simulink model "Nanogrid"  (R2026a)
settings: Solver=VariableStepAuto  StopTime=3
PreLoadFcn:
  | NanogridParam
undefined symbols (not defined in the file): baseLoad, bessSystem, bessVoltage, DiscIntNeverNeededParam, ee_sli_rtmsupport, gcbh, gflInverter, gfmInverter, nanoLoad, PV, PVInverter, ref, solar, solarInsolationChange, Ts
libraries: nesl_utility x51, eeGeneralControl x38, ee_lib x33, fl_lib x24, simulink x20, eeTransforms x13, slpidlib x8, nesl_utility_internal x4, sl_signal_attributes x4, sl_discontinuities x4, eeSinusoidalMeasurementV2 x3, batteryecm_lib x2
(part 1 of 6)
settings Model: Creator=claude-test  LastModifiedBy=claude-test

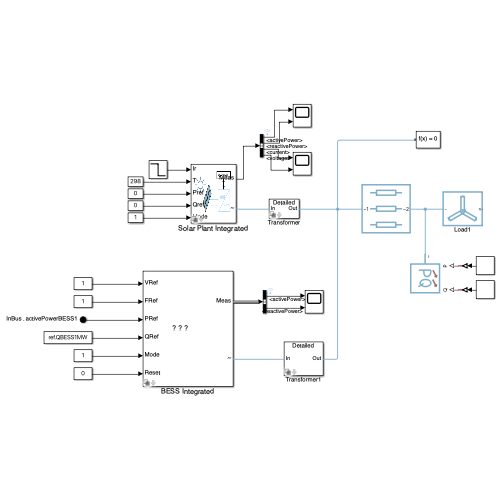
[thumbnail: Simulink's stored preview of the top-level diagram]
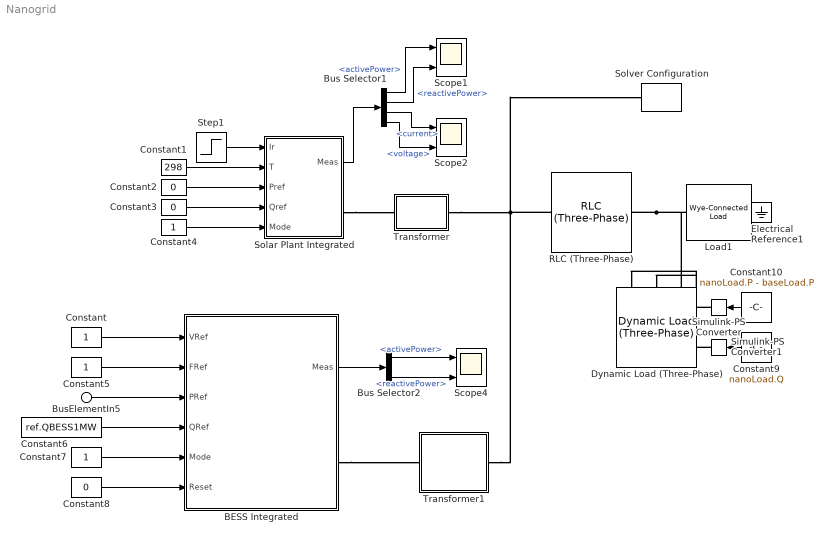
== system Nanogrid ==
  BusElementIn5 : Inport  PortName=InBus  Element=activePowerBESS1
  BESS Integrated : Subsystem  Variant=on  VariantControlMode=label  LabelModeActiveChoice=Detailed  mask(Battery Energy Storage System (BESS)){fidelity=Detailed, bessController=Grid Forming, plantRating=bessSystem.plantRating, Vac=bessSystem.Vac, frequency=bessSystem.frequency, iMaxPU=bessSystem.iMaxPU, efficiency=bessSystem.converterEfficiency, baseVoltageDC=bessSystem.Vdc, filterInductance=bessSystem.filterInductance, filterResistance=bessSystem.filterResistance, maxSOC=bessSystem.maxSOC, minSOC=bessSystem.minSOC, converterFidelity=Average, fSw=bessSystem.switchingFrequency, activeDroop=bessSystem.activeDroop, reactiveDroop=bessSystem.reactiveDroop, maxSOCGFM=0.95, minSOCGFM=0.1, initialSOC=bessSystem.initialSOC, capacityType=Infinite, capacity=1000}
      mask prompts: fidelity "Modeling Option"; bessController "Operating Mode"; plantRating "BESS Rating (kW)"; Vac "Rated AC side voltage (phase-phase RMS) (V)"; frequency "Rated electrical frequency at AC side (Hz)"; iMaxPU "Maximum converter current (pu)"; efficiency "Converter Efficiency (%)"; baseVoltageDC "Voltage on DC side (V)"; filterInductance "Filter inductance (H)"; filterResistance "Filter series resistance (Ohm)"; maxSOC "Maximum  operating SOC"; minSOC "Minimum  operating SOC"; converterFidelity "Converter Fidelity"; fSw "Switching Frequency (kHz)"; activeDroop "Active droop"; reactiveDroop "Reactive droop"; maxSOCGFM "Maximum  operating SOC"; minSOCGFM "Minimum  operating SOC"; initialSOC "Initial SOC"; capacityType "Battery charge capacity"; capacity "Battery capacity (Ah)"
      mask help:
      | This block represents a flexible BESS that can be configured for different operational modes and modeling fidelities. It supports Grid-Following (GFL) and Grid-Forming (GFM) control strategies, along with two fidelity levels:
      |
      | Detailed – captures dynamic control loops and converter behavior for accurate transient analysis.
      | Simplified – optimized for faster simulations while preserving essential system characteristics.
      settings: CopyFcn=set_param(gcbh,'LinkStatus','none');
      mask Help: web('BESS.html')
      mask TypeOptions fidelity: Detailed | Simplified
      mask Callback fidelity:
      | component.mask.fidelitySelection;
      |     fidelity = get_param(gcb,'fidelity');
      |     mode = get_param(gcb,'bessController');
      |     maskObj = Simulink.Mask.get(gcb);
      |     allNames = {maskObj.Parameters.Name};
      |     effIdx = find(strcmp(allNames, 'efficiency'));
      |     tabGFL = maskObj.getDialogControl('cellSimplified');
      |     tabGFM = maskObj.getDialogControl('cellSimplifiedGFM');
      |     if strcmp(fidelity,'Simplified')
      |         maskObj.Parameters(effIdx).Visible = 'on';
      |         if strcmp(mode,'Grid Following')
      |             tabGFL.Visible = 'on';
      |             tabGFM.Visible = 'off';
      |         else
      |             tabGFL.Visible = 'off';
      |             tabGFM.Visible = 'on';
      |         end
      |     else
      |         maskObj.Parameters(effIdx).Visible = 'off';
      |         tabGFL.Visible = 'off';
      |         tabGFM.Visible = 'off';
      |     end
      mask TypeOptions bessController: Grid Following | Grid Forming
      mask Callback bessController:
      | fidelity = get_param(gcb,'fidelity');
      | mode = get_param(gcb,'bessController');
      | if strcmp(fidelity,'Detailed')
      |     component.mask.setBESSController;
      | else
      |     blockPath = [gcb,'/','Simplified'];
      |     component.mask.setBESSController(blockPath);
      | end
      | maskObj = Simulink.Mask.get(gcb);
      | tabGFL = maskObj.getDialogControl('cellSimplified');
      | tabGFM = maskObj.getDialogControl('cellSimplifiedGFM');
      | if strcmp(fidelity,'Simplified')
      |     if strcmp(mode,'Grid Following')
      |         tabGFL.Visible = 'on';
      |         tabGFM.Visible = 'off';
      |     else
      |         tabGFL.Visible = 'off';
      |         tabGFM.Visible = 'on';
      |     end
      | else
      |     tabGFL.Visible = 'off';
      |     tabGFM.Visible = 'off';
      | end
      mask TypeOptions converterFidelity: Detailed/BESS Plant/converterFidelity
      mask Callback converterFidelity:
      | blockPath = [gcb,'/','Detailed','/','BESS Plant','/','Converter'];
      | component.mask.converterFidelity(blockPath);
      mask TypeOptions fSw: Detailed/PV Plant & Controller/PV Plant/fSw
      mask TypeOptions initialSOC: Simplified/Grid Forming/initialSOC
      mask TypeOptions capacityType: Simplified/Grid Forming/capacityType
      mask Callback capacityType: component.mask.configureBatteryCapacity;
      mask TypeOptions capacity: Simplified/Grid Forming/capacity
      mask DialogControl generalDetailed Prompt: General
      mask DialogControl cellDetailed Prompt: Battery
      mask DialogControl configureBattery Prompt: Edit battery parameters
      mask DialogControl configureBattery Callback:
      | blockPath = [gcb,'/','Detailed','/','BESS Plant','/','Battery'] ;
      |     component.mask.openBlock(blockPath);
      mask DialogControl controllerDetailed Prompt: BESS Controller
      mask DialogControl configureBESSController Prompt: Edit BESS Controller
      mask DialogControl configureBESSController Callback:
      | controllerType = get_param(gcb,'bessController');
      |     blockPath = [gcb,'/','Detailed','/','BESS Controller','/',controllerType];
      |     component.mask.openBlock(blockPath);
      mask DialogControl cellSimplified Prompt: Battery
      mask DialogControl configureBatterySimplified Prompt: Edit battery parameters
      mask DialogControl configureBatterySimplified Callback:
      | mode = get_param(gcb,'bessController');
      |     blockPath = [gcb,'/','Simplified','/',mode,'/','Battery'] ;
      |     if strcmp(mode,'Grid Following')
      |         component.mask.openBlock(blockPath);
      |     end
      mask DialogControl converter Prompt: Converter
      mask DialogControl editConverter Prompt: Edit converter parameters
      mask DialogControl editConverter Callback:
      | converterFidelity = get_param(gcb,'converterFidelity');
      | blockPath = [gcb,'/','Detailed','/','BESS Plant','/','Converter','/',converterFidelity,'/','Converter'];
      | component.mask.openBlock(blockPath);
      mask DialogControl cellSimplifiedGFM Prompt: Battery
      mask Display: image('battery_detailed.png');
  Bus Selector1 : BusSelector  OutputSignals=activePower,reactivePower,current,voltage
  Bus Selector2 : BusSelector  OutputSignals=activePower,reactivePower
  Constant{,4..5,7} (4 alike) : Constant
  Constant1 : Constant  Value=298
  Constant10 : Constant  Value=nanoLoad.P - baseLoad.P
  Constant2 : Constant  Value=0
  Constant3 : Constant  Value=0
  Constant6 : Constant  Value=ref.QBESS1MW
  Constant8 : Constant  Value=0
  Constant9 : Constant  Value=nanoLoad.Q
  Dynamic Load (Three-Phase) : ee_lib/Passive/Dynamic Load (Three-Phase)  port_option=ee.enum.threePhasePort.composite  FRated=systemFrequency Hz  Vline_rms_min=7700 V  tau=0.0167 s  Vline_rms_ini=11000 V  Vang_ini=0 deg  gmin=0 S
  Electrical Reference1 : fl_lib/Electrical/Electrical Elements/Electrical Reference
  Load1 : ee_lib/Passive/RLC Assemblies/Wye-Connected Load  port_option=ee.enum.threePhasePort.composite  parameterization=ee.enum.rlc.parameterization.ratedpower  component_structure=ee.enum.rlc.structure.R  component_structure_PQ=ee.enum.rlc.structure.R  R=1 Ohm  L=1e-3 H  C=1e-6 F  VRated=busVoltage V  FRated=systemFrequency Hz  P=baseLoad.P W  Qpos=0 A*V  Qneg=-1e2 A*V  R_parasitic=1e-6 Ohm  G_parasitic=1e-6 1/Ohm  R_parasitic_PQ=1e-6 Ohm  G_parasitic_PQ=1e-6 1/Ohm  Vmag0=busVoltage V  Vang0=0 deg  Freq0=systemFrequency Hz  IL_specify=off  IL_priority=High  IL=[0, 0, 0] A  IL_nominal_specify=off  IL_nominal_value=1  IL_nominal_unit=A  VC_specify=off  VC_priority=High  VC=[0, 0, 0] V  VC_nominal_specify=off  VC_nominal_value=1  VC_nominal_unit=V
  RLC (Three-Phase) : ee_lib/Passive/RLC Assemblies/RLC (Three-Phase)  port_option=ee.enum.threePhasePort.composite  component_structure=ee.enum.rlc.structure.SeriesRL  R=1 Ohm  L=1e-03 H  C=1e-6 F  R_parasitic=0 Ohm  G_parasitic=0 1/Ohm  IL_specify=off  IL_priority=High  IL=[0, 0, 0] A  IL_nominal_specify=off  IL_nominal_value=1  IL_nominal_unit=A  VC_specify=off  VC_priority=High  VC=[0, 0, 0] V  VC_nominal_specify=off  VC_nominal_value=1  VC_nominal_unit=V
  Scope1 : Scope  NumInputPorts=2
      settings: ActiveDisplayYMinimum=-0.88286408189414312  ActiveDisplayYMaximum=1.6939099105793236  DataLoggingVariableName=ScopeData17
  Scope2 : Scope  NumInputPorts=2
      settings: ActiveDisplayYMinimum=-0.88286408189414312  ActiveDisplayYMaximum=1.6939099105793236  DataLoggingVariableName=ScopeData18
  Scope4 : Scope  NumInputPorts=2
      settings: ActiveDisplayYMinimum=-0.88286408189414312  ActiveDisplayYMaximum=1.6939099105793236  DataLoggingVariableName=ScopeData55
  Simulink-PS Converter : nesl_utility/Simulink-PS Converter  PhysicalDomain=network_engine_domain  SubClassName=ps_input  LeftPortType=input  RightPortType=output  PseudoPeriodic=off  Frequencies=[]  NoiseDistribution=none  NoiseParameters=[]  Unit=1  AffineConversion=off  FilteringAndDerivatives=provide  SimscapeFilterOrder=1  InputFilterTimeConstant=0.001  UdotUserProvided=0
  Simulink-PS Converter1 : nesl_utility/Simulink-PS Converter  PhysicalDomain=network_engine_domain  SubClassName=ps_input  LeftPortType=input  RightPortType=output  PseudoPeriodic=off  Frequencies=[]  NoiseDistribution=none  NoiseParameters=[]  Unit=1  AffineConversion=off  FilteringAndDerivatives=provide  SimscapeFilterOrder=1  InputFilterTimeConstant=0.001  UdotUserProvided=0
  Solar Plant Integrated : Subsystem  Variant=on  VariantControlMode=label  LabelModeActiveChoice=Detailed  mask(Solar){fidelity=Detailed, plantRating=PV.plantRating, Vac=PV.Vac, frequency=PV.frequency, iMaxPU=PVInverter.iMaxPU, efficiency=PV.converterEfficiency, baseVoltageDC=PV.baseVoltageDC, nParallel=PV.nParallel, nSeries=30, capacitance=PVInverter.capacitance, filterInductance=PVInverter.filterInductance, filterResistance=PVInverter.filterResistance, panelType=Poly-crystalline, panelRating=PV.panelRating, Isc=PV.Isc, Voc=PV.Voc, irradianceSTC=PV.irradianceSTC, temperatureSTC=PV.temperatureSTC, alpha=PV.alpha, beta=PV.beta, mode=Maximum power point tracking, converterFidelity=Average, fSw=PV.switchingFrequency}
      mask prompts: fidelity "Modeling Option"; plantRating "Solar Plant Rating (kW)"; Vac "Rated AC side voltage (phase-phase RMS) (V)"; frequency "Rated electrical frequency at AC side (Hz)"; iMaxPU "Maximum converter current (pu)"; efficiency "Converter Efficiency (%)"; baseVoltageDC "Voltage on DC side (V)"; nParallel "Number of panels in parallel"; nSeries "Number of panels in series"; capacitance "DC bus capacitance (F)"; filterInductance "Filter inductance (H)"; filterResistance "Filter series resistance (Ohm)"; panelType "Panel Type"; panelRating "Panel Rating (W)"; Isc "Short-circuit current (A)"; Voc "Open-circuit voltage (V)"; irradianceSTC "Irradiance at STC (W/m² )"; temperatureSTC "Temperature at STC (°K)"; alpha "Temperature co-efficient for current (A/°K)"; beta "Temperature co-efficient for voltage (V/°K)"; mode "Operating Mode"; converterFidelity "Converter Fidelity"; fSw "Switching Frequency (kHz)"
      mask help: This block models a Solar PV plant. The detailed variant models MPPT, voltage and current controllers. The simplified variant is based on Anderson's translational equations. Select simplified mode for faster simulation using fixed efficiency and rated power.
      settings: CopyFcn=set_param(gcbh,'LinkStatus','none');
      mask Help: web('SolarPlant.html')
      mask TypeOptions fidelity: Detailed | Simplified
      mask Callback fidelity: component.mask.fidelitySelection;
      mask TypeOptions nParallel: Detailed/PV Plant & Controller/PV Plant/nParallel
      mask TypeOptions nSeries: Detailed/PV Plant & Controller/PV Plant/nSeries
      mask TypeOptions panelType: Poly-crystalline | Mono-crystalline | Cadmium-Telluride | Others
      mask Callback panelType: component.mask.selectSolarPanelType;
      mask TypeOptions mode: Maximum power point tracking | Power reference
      mask Callback mode:
      | % choice = get_param(gcb,'mode');
      | % blockPath = [gcb,'/','Solar','/','Simplified','/','Solar_Plant'];
      | % blockHandle = get_param(blockPath, 'Handle');
      | % if strcmp(choice,'Maximum power point tracking')
      | %     set_param(blockPath,'modelling_option','ModellingOption.maximumPower');
      | % else
      | %     set_param(blockPath,'modelling_option','ModellingOption.powerReference');
      | % end
      mask TypeOptions converterFidelity: Detailed/PV Plant & Controller/PV Plant/converterFidelity
      mask Callback converterFidelity: component.mask.setSwitchingFrequency;
      mask TypeOptions fSw: Detailed/PV Plant & Controller/PV Plant/fSw
      mask DialogControl generalDetailed Prompt: General
      mask DialogControl cellDetailed Prompt: Solar Cell
      mask DialogControl partsCatalog Prompt: Click to choose from parts catalog
      mask DialogControl partsCatalog Callback: component.mask.openParamManager;
      mask DialogControl panelCalculation Prompt: Calculate number of panels
      mask DialogControl panelCalculation Callback: component.mask.setPanelNumber;
      mask DialogControl configureSolarCell Prompt: Edit Solar Cell Parameters
      mask DialogControl configureSolarCell Callback:
      | blockPath = [gcb,'/','Detailed','/','PV Plant & Controller','/','PV Plant','/','PV Array'];
      |     component.mask.openBlock(blockPath);
      mask DialogControl controllerDetailed Prompt: Solar PV Controller
      mask DialogControl configurePVController Prompt: Edit MPPT Controller
      mask DialogControl configurePVController Callback:
      | blockPath = [gcb,'/','Detailed','/','PV Plant & Controller','/','Controller','/','MPPT','/','Solar PV Controller'];
      |     component.mask.openBlock(blockPath);
      mask DialogControl configurePRefControl Prompt: Edit Power Reference Controller
      mask DialogControl configurePRefControl Callback:
      | blockPath = [gcb,'/','Detailed','/','PV Plant & Controller','/','Controller','/','Power Reference','/','Power Reference Controller'];
      |     component.mask.openBlock(blockPath);
      mask DialogControl cellSimplified Prompt: Solar Cell
      mask DialogControl converter Prompt: Converter
      mask DialogControl editConverter Prompt: Edit converter parameters
      mask DialogControl editConverter Callback:
      | converterFidelity = get_param(gcb,'converterFidelity');
      | blockPath = [gcb,'/','Detailed','/','PV Plant & Controller','/','PV Plant','/','Converter','/',converterFidelity,'/','Converter'];
      | component.mask.openBlock(blockPath);
      mask Display: image('solarPlant.png');
  Solver Configuration : nesl_utility/Solver Configuration  PhysicalDomain=network_engine_domain  SubClassName=solver  LeftPortType=input  RightPortType=generic  Tones=[]  Harmonics=[]  SimulateNoise=off  Profile=off  UseLocalSampling=off  EnableSwitchedLinearOptims=on  FrequencyDomain=off  UseCCode=off  RelTol=0.001  AbsTol=0.001  MinStep=1e-09  ToWorkspace=off  RevertToSquareIcSolve=off  NumHomotopyIterations=100  PhasorMode=off  PhasorModeNumHarmonics=1  ConsistencySolver=NEWTON_XTOL_AFTER_FTOL  CanonicalOrdering=UNORDERED  OptimizeIntermediates=UNOPTIMIZED  IndexReductionMethod=None  DoDC=off  ResidualTolerance=1e-09  ConsistencyTolSource=GLOBAL  ConsistencyAbsTol=0.001  ConsistencyRelTol=0.001  ConsistencyTolFactor=1e3  UseLocalSolver=on  LocalSolverChoice=NE_BACKWARD_EULER_ADVANCER  ResolveIndetEquations=off  FunctionEvalNumThread=1  LocalSolverSampleTime=5e-05  DoFixedCost=on  MaxNonlinIter=1  MaxModeIter=2  ComputeImpulses=off  ImpulseIterations=2  LinearAlgebra=Sparse  LinearAlgebraNumThread=0  EquationFormulation=NE_TIME_EF  DelaysMemoryBudget=1024  AutomaticFiltering=off  FilteringTimeConstant=0.001  PartitionStorageMethod=AS_NEEDED  PartitionMemoryBudget=1024  PartitionMethod=ROBUST  MultibodyUseLocalSolver=off  MultibodyLocalSolverChoice=ODE1  MultibodyLocalSolverSampleTime=0.001
  Step1 : Step  Time=solarInsolationChange  InitialValue=1000  FinalValue=800  SampleTime=0
  Transformer : Subsystem  Variant=on  VariantControlMode=label  LabelModeActiveChoice=Detailed  mask{fidelity=Detailed}
      mask prompts: fidelity "Modeling Option"
      mask TypeOptions fidelity: Detailed | Simplified
      mask Callback fidelity:
      | choice = get_param(gcb,'fidelity');
      | switch choice
      |     case 'Detailed'
      |         set_param(gcb, 'LabelModeActiveChoice', 'Detailed');
      |     case 'Simplified'
      |          set_param(gcb, 'LabelModeActiveChoice', 'Simplified');
      |     otherwise
      |         disp('Choose proper variant');
      | end
  Transformer1 : Subsystem  Variant=on  VariantControlMode=label  LabelModeActiveChoice=Detailed  mask{fidelity=Detailed}
      mask prompts: fidelity "Modeling Option"
      mask TypeOptions fidelity: Detailed | Simplified
      mask Callback fidelity:
      | choice = get_param(gcb,'fidelity');
      | switch choice
      |     case 'Detailed'
      |         set_param(gcb, 'LabelModeActiveChoice', 'Detailed');
      |     case 'Simplified'
      |          set_param(gcb, 'LabelModeActiveChoice', 'Simplified');
      |     otherwise
      |         disp('Choose proper variant');
      | end
  wires:
  Constant3/1 -> Solar Plant Integrated/4(Qref)
  Step1/1 -> Solar Plant Integrated/1(Ir)
  Constant2/1 -> Solar Plant Integrated/3(Pref)
  Constant1/1 -> Solar Plant Integrated/2(T)
  Constant4/1 -> Solar Plant Integrated/5(Mode)
  Constant7/1 -> BESS Integrated/5(Mode)
  BESS Integrated/1(Meas) -> Bus Selector2/1
  Constant6/1 -> BESS Integrated/4(QRef)
  Constant/1 -> BESS Integrated/1(VRef)
  BusElementIn5/1 -> BESS Integrated/3(PRef)
  Constant8/1 -> BESS Integrated/6(Reset)
  Bus Selector2/2 -> Scope4/2  "<reactivePower>"
  Bus Selector2/1 -> Scope4/1  "<activePower>"
  Constant5/1 -> BESS Integrated/2(FRef)
  Constant9/1 -> Simulink-PS Converter1/1
  Constant10/1 -> Simulink-PS Converter/1
  Solar Plant Integrated/1(Meas) -> Bus Selector1/1
  Bus Selector1/1 -> Scope1/1  "<activePower>"
  Bus Selector1/2 -> Scope1/2  "<reactivePower>"
  Bus Selector1/3 -> Scope2/1  "<current>"
  Bus Selector1/4 -> Scope2/2  "<voltage>"
  connections:
  Solar Plant Integrated/RConn1 -- Transformer/LConn1
  BESS Integrated/RConn1 -- Transformer1/LConn1
  Electrical Reference1/LConn1 -- Load1/RConn1
  Transformer/RConn1 -- RLC (Three-Phase)/LConn1 -- Solver Configuration/RConn1 -- Transformer1/RConn1
  Simulink-PS Converter/RConn1 -- Dynamic Load (Three-Phase)/LConn2
  Simulink-PS Converter1/RConn1 -- Dynamic Load (Three-Phase)/LConn3
  Load1/LConn1 -- Dynamic Load (Three-Phase)/LConn1 -- RLC (Three-Phase)/RConn1

== system Nanogrid/BESS Integrated ==
  VRef : Inport
  FRef : Inport  Port=2
  PRef : Inport  Port=3
  QRef : Inport  Port=4
  Mode : Inport  Port=5
  Reset : Inport  Port=6
  Detailed : Subsystem  VariantControl=Detailed
  Simplified : Subsystem  Variant=on  VariantControlMode=label  VariantControl=Simplified  LabelModeActiveChoice=Grid Forming
  ~ : PMIOPort  Side=Right
  Meas : Outport

== system Nanogrid/Solar Plant Integrated ==
  Ir : Inport
  T : Inport  Port=2
  Pref : Inport  Port=3
  Qref : Inport  Port=4
  Mode : Inport  Port=5
  Detailed : Subsystem  VariantControl=Detailed
  Simplified : Subsystem  VariantControl=Simplified
  ~ : PMIOPort  Side=Right
  Meas : Outport

== system Nanogrid/Transformer ==
  Detailed : Subsystem  VariantControl=Detailed
  Simplified : Subsystem  VariantControl=Simplified  mask{windingRatio=690/6600}
      mask prompts: windingRatio "Winding ratio"
      mask DialogControl Container4 Prompt: General
  In : PMIOPort  Side=Left
  Out : PMIOPort  Port=2  Side=Right

== system Nanogrid/Transformer1 ==
  Detailed : Subsystem  VariantControl=Detailed
  Simplified : Subsystem  VariantControl=Simplified  mask{windingRatio=690/6600}
      mask prompts: windingRatio "Winding ratio"
      mask DialogControl Container4 Prompt: General
  In : PMIOPort  Side=Left
  Out : PMIOPort  Port=2  Side=Right

== system Nanogrid/BESS Integrated/Detailed ==
  note: Plant
  note: Controller
  VRef : Inport
  FRef : Inport  Port=2
  PRef : Inport  Port=3
  QRef : Inport  Port=4
  Mode : Inport  Port=5
  Reset : Inport  Port=6
  BESS Controller : Subsystem  Variant=on  VariantControlMode=label  LabelModeActiveChoice=Grid Forming
  BESS Plant : Subsystem  mask(BESS Plant){converterFidelity=Average, fSw=fSw, ratedVoltage=Vac}
      mask prompts: converterFidelity "Converter Fidelity"; fSw "Switching Frequency (kHz)"; ratedVoltage "Rated voltage on AC side (V)"
      mask help: This block represents the physical interface between the battery and the power converter. It models the electrical and dynamic characteristics of the battery system connected to a converter, while expecting an external control signal for operation
      settings: CopyFcn=set_param(gcbh,'LinkStatus','none');
      mask TypeOptions converterFidelity: Converter/converterFidelity
      mask Callback converterFidelity: component.mask.converterFidelityPlant;
      mask TypeOptions fSw: Converter/fSw
      mask DialogControl Container4 Prompt: General
      mask DialogControl editBattery Prompt: Edit battery parameters
      mask DialogControl editBattery Callback:
      | blockPath = [gcb,'/','Battery'];
      | component.mask.openBlock(blockPath);
      mask DialogControl editConverter Prompt: Edit converter parameters
      mask DialogControl editConverter Callback:
      | converterFidelity = get_param(gcb,'converterFidelity');
      | blockPath = [gcb,'/','Converter','/',converterFidelity,'/','Converter'];
      | component.mask.openBlock(blockPath);
      mask Display: image('battery.png');
  Filter & Measurements : Subsystem
  ~ : PMIOPort  Side=Right
  Meas : Outport
  wires:
  BESS Plant/1(SOC) -> Filter & Measurements/1(SOC)
  FRef/1 -> BESS Controller/2(FRef)
  Mode/1 -> BESS Controller/5(Mode)
  PRef/1 -> BESS Controller/3(PRef)
  Filter & Measurements/1(VIBus) -> BESS Controller/7(VIBus)
  QRef/1 -> BESS Controller/4(QRef)
  VRef/1 -> BESS Controller/1(VRef)
  Reset/1 -> BESS Controller/6(Reset)
  Filter & Measurements/2(Meas) -> Meas/1
  BESS Controller/1(mabc) -> BESS Plant/1(mabc)
  connections:
  Filter & Measurements/RConn1 -- ~/RConn1
  BESS Plant/RConn1 -- Filter & Measurements/LConn1

== system Nanogrid/BESS Integrated/Simplified ==
  VRef : Inport
  FRef : Inport  Port=2
  PRef : Inport  Port=3
  QRef : Inport  Port=4
  Mode : Inport  Port=5
  Reset : Inport  Port=6
  Grid Following : Subsystem  VariantControl=Grid Following  mask(BESS GFL Simplified){plantRating=plantRating, Vac=Vac, frequency=frequency, iMaxPU=iMaxPU, efficiency=efficiency, bessVoltage=baseVoltageDC, maxSOC=maxSOC, minSOC=minSOC}
      mask prompts: plantRating "BESS Rating (kW)"; Vac "Rated AC side voltage (phase-phase RMS) (V)"; frequency "Rated electrical frequency at AC side (Hz)"; iMaxPU "Maximum converter current (pu)"; efficiency "Converter Efficiency (%)"; bessVoltage "Nominal BESS voltage (V)"; maxSOC "Maximum operating SOC"; minSOC "Minimum operating SOC"
      mask help: This block models a BESS that synchronizes with grid voltage and frequency using simplified control representation. This block is designed for computational efficiency, ideal for system-level studies in strong grid conditions where detailed transient behavior is less critical.
      settings: CopyFcn=set_param(gcbh,'LinkStatus','none');
      mask DialogControl generalDetailed Prompt: General
      mask DialogControl Container5 Prompt: Battery
      mask DialogControl editBattery Prompt: Edit battery parameters
      mask DialogControl editBattery Callback:
      | blockPath = [gcb,'/','Battery'] ;
      | component.mask.openBlock(blockPath);
  Grid Forming : Subsystem  VariantControl=Grid Forming  mask(BESS GFM Simplified){plantRating=plantRating, Vac=Vac, frequency=frequency, Vdc=baseVoltageDC, iMaxPU=iMaxPU, efficiency=efficiency, activeDroop=activeDroop, reactiveDroop=reactiveDroop, initialSOC=initialSOC, maxSOC=0.95, minSOC=0.1, capacityType=Infinite, capacity=capacity}
      mask prompts: plantRating "BESS Rating (kW)"; Vac "Rated AC side voltage (phase-phase RMS) (V)"; frequency "Rated electrical frequency at AC side (Hz)"; Vdc "Nominal DC bus voltage (V)"; iMaxPU "Maximum converter current (pu)"; efficiency "Converter Efficiency (%)"; activeDroop "Active droop"; reactiveDroop "Reactive droop"; initialSOC "Initial SOC"; maxSOC "Maximum operating SOC"; minSOC "Minimum operating SOC"; capacityType "Battery charge capacity"; capacity "Battery capacity (Ah)"
      mask help: This block models a BESS with generating voltage and frequency reference capabilities. It is optimized for faster simulations while maintaining essential grid-forming behavior, making it suitable for large-scale stability studies or planning scenarios where detailed converter dynamics are not required.
      settings: CopyFcn=set_param(gcbh,'LinkStatus','none');
      mask TypeOptions capacityType: Fixed | Infinite
      mask Callback capacityType: component.mask.configureBatteryCapacity;
      mask DialogControl generalDetailed Prompt: General
      mask DialogControl Container5 Prompt: Battery
  ~ : PMIOPort  Side=Right
  Meas : Outport

== system Nanogrid/Solar Plant Integrated/Detailed ==
  Ir : Inport
  T : Inport  Port=2
  Pref : Inport  Port=3
  Qref : Inport  Port=4
  Mode : Inport  Port=5
  L Filter2 : ee_lib/Passive/RLC Assemblies/RLC (Three-Phase)  port_option=ee.enum.threePhasePort.composite  component_structure=ee.enum.rlc.structure.SeriesRL  R=filterResistance Ohm  L=filterInductance H  C=1e-6 F  R_parasitic=0 Ohm  G_parasitic=0 1/Ohm  IL_specify=on  IL_priority=None  IL=[0, 0, 0] A  IL_nominal_specify=off  IL_nominal_value=1  IL_nominal_unit=A  VC_specify=off  VC_priority=High  VC=[0, 0, 0] V  VC_nominal_specify=off  VC_nominal_value=1  VC_nominal_unit=V
  Measurements : Subsystem
  PV Plant & Controller : Subsystem
  Terminator : Terminator
  ~ : PMIOPort  Side=Right
  Out Bus Element23 : Outport  PortName=Meas  Element=activePower
  Out Bus Element1 : Outport  PortName=Meas  Element=reactivePower
  Out Bus Element2 : Outport  PortName=Meas  Element=voltage
  Out Bus Element3 : Outport  PortName=Meas  Element=current
  wires:
  Measurements/2(Q) -> Out Bus Element1/1
  Measurements/4(I) -> Out Bus Element3/1, PV Plant & Controller/5(Iabc)
  Qref/1 -> PV Plant & Controller/3(Qref)
  Ir/1 -> PV Plant & Controller/1(Insolation)
  Measurements/3(V) -> Out Bus Element2/1, PV Plant & Controller/4(Vabc)
  Measurements/1(P) -> Out Bus Element23/1
  T/1 -> Terminator/1
  Pref/1 -> PV Plant & Controller/2(Pref)
  Mode/1 -> PV Plant & Controller/6(Mode)
  connections:
  L Filter2/RConn1 -- Measurements/LConn1
  L Filter2/LConn1 -- PV Plant & Controller/RConn1
  Measurements/RConn1 -- ~/RConn1

== system Nanogrid/Solar Plant Integrated/Simplified ==
  Ir : Inport
  T : Inport  Port=2
  Pref : Inport  Port=3
  Qref : Inport  Port=4
  Mode : Inport  Port=5
  Measurements : Subsystem
  Simulink-PS Converter{,1..4} (5 alike) : nesl_utility/Simulink-PS Converter  PhysicalDomain=network_engine_domain  SubClassName=ps_input  LeftPortType=input  RightPortType=output  PseudoPeriodic=off  Frequencies=[]  NoiseDistribution=none  NoiseParameters=[]  Unit=1  AffineConversion=off  FilteringAndDerivatives=provide  SimscapeFilterOrder=1  InputFilterTimeConstant=0.001  UdotUserProvided=0
  solar_plant : custom_lib/solar_plant  port_option=ee.enum.threePhasePort.composite  FRated=frequency Hz  VRated=Vac V  PlantRating=plantRating kW  modelling_option=ModellingOption.powerReference  Vdc=2*Vac*sqrt(2/3) V  IMaxPU=iMaxPU  efficiency=efficiency  IrRef=irradianceSTC W/m^2  T=temperatureSTC K  PVTech=PanelTechnology.polycrystallinePanel  PanelRating=panelRating W  VocRef=Voc V  IscRef=Isc A  alpha=alpha 1/K  beta=beta 1/K  delta=0.111
      settings: SourceProductName=Microgrids
  ~ : PMIOPort  Side=Right
  Bus Element Out : Outport  PortName=Meas  Element=activePower
  BusElementOut : Outport  PortName=Meas  Element=reactivePower
  BusElementOut1 : Outport  PortName=Meas  Element=voltage
  BusElementOut2 : Outport  PortName=Meas  Element=current
  wires:
  Measurements/4(I) -> BusElementOut2/1
  Measurements/3(V) -> BusElementOut1/1
  Measurements/2(Q) -> BusElementOut/1
  Measurements/1(P) -> Bus Element Out/1
  Ir/1 -> Simulink-PS Converter/1
  T/1 -> Simulink-PS Converter1/1
  Pref/1 -> Simulink-PS Converter2/1
  Qref/1 -> Simulink-PS Converter3/1
  Mode/1 -> Simulink-PS Converter4/1
  connections:
  solar_plant/LConn5 -- Simulink-PS Converter3/RConn1
  solar_plant/LConn3 -- Simulink-PS Converter4/RConn1
  ~/RConn1 -- Measurements/RConn1
  Measurements/LConn1 -- solar_plant/RConn1
  Simulink-PS Converter/RConn1 -- solar_plant/LConn1
  Simulink-PS Converter1/RConn1 -- solar_plant/LConn2
  solar_plant/LConn4 -- Simulink-PS Converter2/RConn1

== system Nanogrid/Transformer/Detailed ==
  Two-Winding Transformer (Three-Phase)2 : ee_lib/Passive/Transformers/Two-Winding Transformer (Three-Phase)  SRated=PV.transformerVA A*V  FRated=systemFrequency Hz  Winding1Connection=ee.enum.windingconnection.Yg  VRated1=690 V  Winding2Connection=ee.enum.windingconnection.Yg  VRated2=11000 V  CoreType=ee.enum.coretype.threelimb  pu_Rw1=0.01  pu_Rw2=0.01  leakage_reactance_option=ee.enum.transformer_leakage.include  pu_Xl1=0.05  pu_Xl2=0.05  magnetizing_resistance_option=ee.enum.transformer_magnetizingResistance.exclude  pu_Rm=500  magnetizing_reactance_option=ee.enum.transformer_magnetizingReactance.exclude  saturation_option=ee.enum.transformer_saturation.exclude  pu_Xm=500  current_data=[0, .002, 1, 2]  magnetic_flux_data=[0, 1.2, 1.5, 1.51]  pu_X0=0.5  i1_specify=off  i1_priority=None  i1=[0, 0, 0] A  i1_nominal_specify=off  i1_nominal_value=1  i1_nominal_unit=A  i2_specify=off  i2_priority=None  i2=[0, 0, 0] A  i2_nominal_specify=off  i2_nominal_value=1  i2_nominal_unit=A  phi_specify=off  phi_priority=None  phi=[0, 0, 0]  phi_nominal_specify=off  phi_nominal_value=1  phi_nominal_unit=1
  In : PMIOPort  Side=Left
  Out : PMIOPort  Port=2  Side=Right
  connections:
  Two-Winding Transformer (Three-Phase)2/LConn1 -- In/RConn1
  Two-Winding Transformer (Three-Phase)2/RConn1 -- Out/RConn1

== system Nanogrid/Transformer/Simplified ==
  Electrical Reference : fl_lib/Electrical/Electrical Elements/Electrical Reference
  Electrical Reference1 : fl_lib/Electrical/Electrical Elements/Electrical Reference
  Ideal Transformer : fl_lib/Electrical/Electrical Elements/Ideal Transformer  n=windingRatio  i1_specify=off  i1_priority=None  i1=0 A  i1_nominal_specify=off  i1_nominal_value=1  i1_nominal_unit=A  v1_specify=off  v1_priority=None  v1=0 V  v1_nominal_specify=off  v1_nominal_value=1  v1_nominal_unit=V  i2_specify=off  i2_priority=None  i2=0 A  i2_nominal_specify=off  i2_nominal_value=1  i2_nominal_unit=A  v2_specify=off  v2_priority=None  v2=0 V  v2_nominal_specify=off  v2_nominal_value=1  v2_nominal_unit=V
  Ideal Transformer1 : fl_lib/Electrical/Electrical Elements/Ideal Transformer  n=windingRatio  i1_specify=off  i1_priority=None  i1=0 A  i1_nominal_specify=off  i1_nominal_value=1  i1_nominal_unit=A  v1_specify=off  v1_priority=None  v1=0 V  v1_nominal_specify=off  v1_nominal_value=1  v1_nominal_unit=V  i2_specify=off  i2_priority=None  i2=0 A  i2_nominal_specify=off  i2_nominal_value=1  i2_nominal_unit=A  v2_specify=off  v2_priority=None  v2=0 V  v2_nominal_specify=off  v2_nominal_value=1  v2_nominal_unit=V
  Ideal Transformer2 : fl_lib/Electrical/Electrical Elements/Ideal Transformer  n=windingRatio  i1_specify=off  i1_priority=None  i1=0 A  i1_nominal_specify=off  i1_nominal_value=1  i1_nominal_unit=A  v1_specify=off  v1_priority=None  v1=0 V  v1_nominal_specify=off  v1_nominal_value=1  v1_nominal_unit=V  i2_specify=off  i2_priority=None  i2=0 A  i2_nominal_specify=off  i2_nominal_value=1  i2_nominal_unit=A  v2_specify=off  v2_priority=None  v2=0 V  v2_nominal_specify=off  v2_nominal_value=1  v2_nominal_unit=V
  Phase Splitter : ee_lib/Connectors & References/Phase Splitter
  Phase Splitter1 : ee_lib/Connectors & References/Phase Splitter
  RLC (Three-Phase) : ee_lib/Passive/RLC Assemblies/RLC (Three-Phase)  Commented=through  port_option=ee.enum.threePhasePort.composite  component_structure=ee.enum.rlc.structure.R  R=1e-9 Ohm  L=1e-3 H  C=1e-6 F  R_parasitic=0 Ohm  G_parasitic=0 1/Ohm  IL_specify=off  IL_priority=High  IL=[0, 0, 0] A  IL_nominal_specify=off  IL_nominal_value=1  IL_nominal_unit=A  VC_specify=off  VC_priority=High  VC=[0, 0, 0] V  VC_nominal_specify=off  VC_nominal_value=1  VC_nominal_unit=V
  In : PMIOPort  Side=Left
  Out : PMIOPort  Port=2  Side=Right
  connections:
  Ideal Transformer/RConn2 -- Electrical Reference1/LConn1 -- Ideal Transformer1/RConn2 -- Ideal Transformer2/RConn2
  Phase Splitter/RConn3 -- Ideal Transformer2/LConn1
  Phase Splitter/RConn2 -- Ideal Transformer1/LConn1
  Phase Splitter/RConn1 -- Ideal Transformer/LConn1
  Ideal Transformer/LConn2 -- Electrical Reference/LConn1 -- Ideal Transformer1/LConn2 -- Ideal Transformer2/LConn2
  Phase Splitter/LConn1 -- In/RConn1
  Phase Splitter1/LConn1 -- RLC (Three-Phase)/LConn1
  Ideal Transformer/RConn1 -- Phase Splitter1/RConn1
  Ideal Transformer2/RConn1 -- Phase Splitter1/RConn3
  Ideal Transformer1/RConn1 -- Phase Splitter1/RConn2
  RLC (Three-Phase)/RConn1 -- Out/RConn1

== system Nanogrid/Transformer1/Detailed ==
  Two-Winding Transformer (Three-Phase)1 : ee_lib/Passive/Transformers/Two-Winding Transformer (Three-Phase)  SRated=bessSystem.transformerVA A*V  FRated=systemFrequency Hz  Winding1Connection=ee.enum.windingconnection.Yg  VRated1=690 V  Winding2Connection=ee.enum.windingconnection.Yg  VRated2=11000 V  CoreType=ee.enum.coretype.threelimb  pu_Rw1=0.01  pu_Rw2=0.01  leakage_reactance_option=ee.enum.transformer_leakage.include  pu_Xl1=0.05  pu_Xl2=0.05  magnetizing_resistance_option=ee.enum.transformer_magnetizingResistance.include  pu_Rm=500  magnetizing_reactance_option=ee.enum.transformer_magnetizingReactance.include  saturation_option=ee.enum.transformer_saturation.exclude  pu_Xm=500  current_data=[0, .002, 1, 2]  magnetic_flux_data=[0, 1.2, 1.5, 1.51]  pu_X0=0.5  i1_specify=off  i1_priority=None  i1=[0, 0, 0] A  i1_nominal_specify=off  i1_nominal_value=1  i1_nominal_unit=A  i2_specify=off  i2_priority=None  i2=[0, 0, 0] A  i2_nominal_specify=off  i2_nominal_value=1  i2_nominal_unit=A  phi_specify=off  phi_priority=None  phi=[0, 0, 0]  phi_nominal_specify=off  phi_nominal_value=1  phi_nominal_unit=1
  In : PMIOPort  Side=Left
  Out : PMIOPort  Port=2  Side=Right
  connections:
  Two-Winding Transformer (Three-Phase)1/LConn1 -- In/RConn1
  Two-Winding Transformer (Three-Phase)1/RConn1 -- Out/RConn1

== system Nanogrid/Transformer1/Simplified ==
  Electrical Reference : fl_lib/Electrical/Electrical Elements/Electrical Reference
  Electrical Reference1 : fl_lib/Electrical/Electrical Elements/Electrical Reference
  Ideal Transformer : fl_lib/Electrical/Electrical Elements/Ideal Transformer  n=windingRatio  i1_specify=off  i1_priority=None  i1=0 A  i1_nominal_specify=off  i1_nominal_value=1  i1_nominal_unit=A  v1_specify=off  v1_priority=None  v1=0 V  v1_nominal_specify=off  v1_nominal_value=1  v1_nominal_unit=V  i2_specify=off  i2_priority=None  i2=0 A  i2_nominal_specify=off  i2_nominal_value=1  i2_nominal_unit=A  v2_specify=off  v2_priority=None  v2=0 V  v2_nominal_specify=off  v2_nominal_value=1  v2_nominal_unit=V
  Ideal Transformer1 : fl_lib/Electrical/Electrical Elements/Ideal Transformer  n=windingRatio  i1_specify=off  i1_priority=None  i1=0 A  i1_nominal_specify=off  i1_nominal_value=1  i1_nominal_unit=A  v1_specify=off  v1_priority=None  v1=0 V  v1_nominal_specify=off  v1_nominal_value=1  v1_nominal_unit=V  i2_specify=off  i2_priority=None  i2=0 A  i2_nominal_specify=off  i2_nominal_value=1  i2_nominal_unit=A  v2_specify=off  v2_priority=None  v2=0 V  v2_nominal_specify=off  v2_nominal_value=1  v2_nominal_unit=V
  Ideal Transformer2 : fl_lib/Electrical/Electrical Elements/Ideal Transformer  n=windingRatio  i1_specify=off  i1_priority=None  i1=0 A  i1_nominal_specify=off  i1_nominal_value=1  i1_nominal_unit=A  v1_specify=off  v1_priority=None  v1=0 V  v1_nominal_specify=off  v1_nominal_value=1  v1_nominal_unit=V  i2_specify=off  i2_priority=None  i2=0 A  i2_nominal_specify=off  i2_nominal_value=1  i2_nominal_unit=A  v2_specify=off  v2_priority=None  v2=0 V  v2_nominal_specify=off  v2_nominal_value=1  v2_nominal_unit=V
  Phase Splitter : ee_lib/Connectors & References/Phase Splitter
  Phase Splitter1 : ee_lib/Connectors & References/Phase Splitter
  In : PMIOPort  Side=Left
  Out : PMIOPort  Port=2  Side=Right
  connections:
  Ideal Transformer/RConn2 -- Electrical Reference1/LConn1 -- Ideal Transformer1/RConn2 -- Ideal Transformer2/RConn2
  Phase Splitter/RConn3 -- Ideal Transformer2/LConn1
  Phase Splitter/RConn2 -- Ideal Transformer1/LConn1
  Phase Splitter/RConn1 -- Ideal Transformer/LConn1
  Ideal Transformer/LConn2 -- Electrical Reference/LConn1 -- Ideal Transformer1/LConn2 -- Ideal Transformer2/LConn2
  Phase Splitter/LConn1 -- In/RConn1
  Phase Splitter1/LConn1 -- Out/RConn1
  Ideal Transformer/RConn1 -- Phase Splitter1/RConn1
  Ideal Transformer2/RConn1 -- Phase Splitter1/RConn3
  Ideal Transformer1/RConn1 -- Phase Splitter1/RConn2
